simulink model "TEP_Final_NoScript"  (R2024a)
settings: Solver=FixedStepAuto  StartTime=0.0  StopTime=10  FixedStep=1/3600  RelTol=1e-3
model workspace (MAT data in the model file):
  AD : Simulink.Parameter (value not decoded)
  AG : Simulink.Parameter (value not decoded)
  AH : Simulink.Parameter (value not decoded)
  AV : Simulink.Parameter (value not decoded)
  AVP : Simulink.Parameter (value not decoded)
  BCHL : Simulink.Parameter (value not decoded)
  BCHV : Simulink.Parameter (value not decoded)
  BD : Simulink.Parameter (value not decoded)
  BG : Simulink.Parameter (value not decoded)
  BH : Simulink.Parameter (value not decoded)
  BVP : Simulink.Parameter (value not decoded)
  CD : Simulink.Parameter (value not decoded)
  CG : Simulink.Parameter (value not decoded)
  CH : Simulink.Parameter (value not decoded)
  CVP : Simulink.Parameter (value not decoded)
  XMW : Simulink.Parameter (value not decoded)
  XNS : Simulink.Parameter (value not decoded)
  XNSE : Simulink.Parameter (value not decoded)
symbols that are objects in the model workspace (value not decoded): AD, AG, AH, AV, AVP, BD, BG, BH, BVP, CD, CG, CH, CVP, XMW, XNS, XNSE
undefined symbols (not defined in the file or in its folder): magnitude, msgbox, SETPT, XMEAS, XMV
libraries: mylib x360, dspindex x28
(part 10 of 14)

== system TEP_Final_NoScript/Subsystem/Braatz/ 10/CONTROL 6 ==
  SETPT(6) : Inport
  XMEAS : Inport  Port=2
  Constant1 : Constant  Value=GAIN6
  Constant2 : Constant  Value=HIGH6
  Constant3 : Constant  Value=SI6
  Constant4 : Constant  Value=XMV6_0
  P Control : Subsystem
  Sampling interval : mylib/Braatz Control/Sampling interval  SystemSampleTime=-1  VariantActivationTime=update diagram  AllowFlexibleInterface=on  Latency=0  AutoFrameSizeCalculation=off
      settings: SourceProductName=TEP Library
  XMV(6) : Outport  VectorParamsAs1DForOutWhenUnconnected=off
  wires:
  Constant2/1 -> P Control/4(High Limit)
  Constant1/1 -> P Control/2(GAIN)
  SETPT(6)/1 -> P Control/1(SETPT)
  P Control/1(XMV_NEW) -> XMV(6)/1
  Sampling interval/1 -> P Control/Action
  Constant3/1 -> Sampling interval/1
  XMEAS/1 -> P Control/3(XMEAS)
  Constant4/1 -> P Control/5(XMV_0)

== system TEP_Final_NoScript/Subsystem/Braatz/ 2/CONTROL 13 ==
  XMEAS(23) : Inport
  Constant : Constant  Value=SETPT13
  Constant1 : Constant  Value=GAIN13
  Constant2 : Constant  Value=TAUI13
  Constant3 : Constant  Value=HIGH13
  Constant5 : Constant  Value=SI13
  Constant6 : Constant  Value=HIGH3
  PI Control Setpoint : mylib/Braatz Control/PI Control Setpoint  SystemSampleTime=-1  VariantActivationTime=update diagram  AllowFlexibleInterface=on  Latency=0  AutoFrameSizeCalculation=off
      settings: SourceProductName=TEP Library
  SETPT_0 : Constant  Value=SETPT3
  Sampling interval : mylib/Braatz Control/Sampling interval  SystemSampleTime=-1  VariantActivationTime=update diagram  AllowFlexibleInterface=on  Latency=0  AutoFrameSizeCalculation=off
      settings: SourceProductName=TEP Library
  SETPT(3) : Outport  VectorParamsAs1DForOutWhenUnconnected=off
  wires:
  Sampling interval/1 -> PI Control Setpoint/Action
  Constant/1 -> PI Control Setpoint/1
  XMEAS(23)/1 -> PI Control Setpoint/2
  PI Control Setpoint/1 -> SETPT(3)/1
  Constant2/1 -> PI Control Setpoint/7
  Constant5/1 -> PI Control Setpoint/6, Sampling interval/1
  Constant1/1 -> PI Control Setpoint/5
  Constant3/1 -> PI Control Setpoint/3
  Constant6/1 -> PI Control Setpoint/4
  SETPT_0/1 -> PI Control Setpoint/8

== system TEP_Final_NoScript/Subsystem/Braatz/ 2/CONTROL 3 ==
  XMEAS(1) : Inport
  SETPT(3) : Inport  Port=2
  Constant1 : Constant  Value=GAIN3
  Constant2 : Constant  Value=HIGH3
  Constant3 : Constant  Value=SI3
  Constant4 : Constant  Value=XMV3_0
  Display2 : Display
  P Control : mylib/Braatz Control/P Control  SystemSampleTime=-1  VariantActivationTime=update diagram  AllowFlexibleInterface=on  Latency=0  AutoFrameSizeCalculation=off
      settings: SourceProductName=TEP Library
  Sampling interval : mylib/Braatz Control/Sampling interval  SystemSampleTime=-1  VariantActivationTime=update diagram  AllowFlexibleInterface=on  Latency=0  AutoFrameSizeCalculation=off
      settings: SourceProductName=TEP Library
  XMV(3) : Outport
  wires:
  Constant2/1 -> P Control/4
  Constant1/1 -> P Control/2
  XMEAS(1)/1 -> Display2/1, P Control/3
  Sampling interval/1 -> P Control/Action
  Constant3/1 -> Sampling interval/1
  Constant4/1 -> P Control/5
  P Control/1 -> XMV(3)/1
  SETPT(3)/1 -> P Control/1

== system TEP_Final_NoScript/Subsystem/Braatz/ 3/CONTROL 17 ==
  XMEAS(8) : Inport
  Constant : Constant  Value=SETPT17
  Constant1 : Constant  Value=GAIN17
  Constant2 : Constant  Value=TAUI17
  Constant3 : Constant  Value=HIGH17
  Constant4 : Constant  Value=SETPT4
  Constant5 : Constant  Value=SI17
  Constant6 : Constant  Value=HIGH4
  PI Control Setpoint : mylib/Braatz Control/PI Control Setpoint  SystemSampleTime=-1  VariantActivationTime=update diagram  AllowFlexibleInterface=on  Latency=0  AutoFrameSizeCalculation=off
      settings: SourceProductName=TEP Library
  Sampling interval : mylib/Braatz Control/Sampling interval  SystemSampleTime=-1  VariantActivationTime=update diagram  AllowFlexibleInterface=on  Latency=0  AutoFrameSizeCalculation=off
      settings: SourceProductName=TEP Library
  SETPT(4) : Outport  VectorParamsAs1DForOutWhenUnconnected=off
  wires:
  Sampling interval/1 -> PI Control Setpoint/Action
  Constant/1 -> PI Control Setpoint/1
  XMEAS(8)/1 -> PI Control Setpoint/2
  PI Control Setpoint/1 -> SETPT(4)/1
  Constant5/1 -> PI Control Setpoint/6, Sampling interval/1
  Constant3/1 -> PI Control Setpoint/3
  Constant6/1 -> PI Control Setpoint/4
  Constant1/1 -> PI Control Setpoint/5
  Constant2/1 -> PI Control Setpoint/7
  Constant4/1 -> PI Control Setpoint/8

== system TEP_Final_NoScript/Subsystem/Braatz/ 3/CONTROL 4 ==
  XMEAS(4) : Inport
  SETPT(4) : Inport  Port=2
  Constant1 : Constant  Value=GAIN4
  Constant2 : Constant  Value=HIGH4
  Constant3 : Constant  Value=SI4
  Constant4 : Constant  Value=XMV4_0
  P Control : mylib/Braatz Control/P Control  SystemSampleTime=-1  VariantActivationTime=update diagram  AllowFlexibleInterface=on  Latency=0  AutoFrameSizeCalculation=off
      settings: SourceProductName=TEP Library
  Sampling interval : mylib/Braatz Control/Sampling interval  SystemSampleTime=-1  VariantActivationTime=update diagram  AllowFlexibleInterface=on  Latency=0  AutoFrameSizeCalculation=off
      settings: SourceProductName=TEP Library
  XMV(4) : Outport  VectorParamsAs1DForOutWhenUnconnected=off
  wires:
  SETPT(4)/1 -> P Control/1
  P Control/1 -> XMV(4)/1
  Sampling interval/1 -> P Control/Action
  Constant3/1 -> Sampling interval/1
  XMEAS(4)/1 -> P Control/3
  Constant1/1 -> P Control/2
  Constant4/1 -> P Control/5
  Constant2/1 -> P Control/4

== system TEP_Final_NoScript/Subsystem/Braatz/ 4/CONTROL 5 ==
  XMEAS(5) : Inport
  Constant1 : Constant  Value=GAIN5
  Constant2 : Constant  Value=HIGH5
  Constant3 : Constant  Value=SI5
  Constant4 : Constant  Value=SETPT5
  Constant5 : Constant  Value=TAUI5
  Constant6 : Constant  Value=XMV5_0
  PI Control : mylib/Braatz Control/PI Control  SystemSampleTime=-1  VariantActivationTime=update diagram  AllowFlexibleInterface=on  Latency=0  AutoFrameSizeCalculation=off
      settings: SourceProductName=TEP Library
  Sampling interval : mylib/Braatz Control/Sampling interval  SystemSampleTime=-1  VariantActivationTime=update diagram  AllowFlexibleInterface=on  Latency=0  AutoFrameSizeCalculation=off
      settings: SourceProductName=TEP Library
  XMV(5) : Outport  VectorParamsAs1DForOutWhenUnconnected=off
  wires:
  Constant2/1 -> PI Control/3
  Constant1/1 -> PI Control/4
  XMEAS(5)/1 -> PI Control/2
  PI Control/1 -> XMV(5)/1
  Sampling interval/1 -> PI Control/Action
  Constant3/1 -> PI Control/5, Sampling interval/1
  Constant4/1 -> PI Control/1
  Constant5/1 -> PI Control/6
  Constant6/1 -> PI Control/7

== system TEP_Final_NoScript/Subsystem/Braatz/ 5/CONTROL 7 ==
  XMEAS(12) : Inport
  Constant1 : Constant  Value=GAIN7
  Constant2 : Constant  Value=HIGH7
  Constant3 : Constant  Value=SI7
  Constant4 : Constant  Value=SETPT7
  Constant5 : Constant  Value=XMV7_0
  P Control : mylib/Braatz Control/P Control  SystemSampleTime=-1  VariantActivationTime=update diagram  AllowFlexibleInterface=on  Latency=0  AutoFrameSizeCalculation=off
      settings: SourceProductName=TEP Library
  Sampling interval : mylib/Braatz Control/Sampling interval  SystemSampleTime=-1  VariantActivationTime=update diagram  AllowFlexibleInterface=on  Latency=0  AutoFrameSizeCalculation=off
      settings: SourceProductName=TEP Library
  XMV(7) : Outport  VectorParamsAs1DForOutWhenUnconnected=off
  wires:
  P Control/1 -> XMV(7)/1
  Sampling interval/1 -> P Control/Action
  Constant3/1 -> Sampling interval/1
  Constant4/1 -> P Control/1
  Constant2/1 -> P Control/4
  XMEAS(12)/1 -> P Control/3
  Constant1/1 -> P Control/2
  Constant5/1 -> P Control/5

== system TEP_Final_NoScript/Subsystem/Braatz/ 6/CONTROL 8 ==
  XMEAS(15) : Inport
  Constant1 : Constant  Value=GAIN8
  Constant2 : Constant  Value=HIGH8
  Constant3 : Constant  Value=SI8
  Constant4 : Constant  Value=SETPT8
  Constant5 : Constant  Value=XMV8_0
  P Control : mylib/Braatz Control/P Control  SystemSampleTime=-1  VariantActivationTime=update diagram  AllowFlexibleInterface=on  Latency=0  AutoFrameSizeCalculation=off
      settings: SourceProductName=TEP Library
  Sampling interval : mylib/Braatz Control/Sampling interval  SystemSampleTime=-1  VariantActivationTime=update diagram  AllowFlexibleInterface=on  Latency=0  AutoFrameSizeCalculation=off
      settings: SourceProductName=TEP Library
  XMV(8) : Outport  VectorParamsAs1DForOutWhenUnconnected=off
  wires:
  P Control/1 -> XMV(8)/1
  Sampling interval/1 -> P Control/Action
  Constant3/1 -> Sampling interval/1
  Constant4/1 -> P Control/1
  Constant2/1 -> P Control/4
  XMEAS(15)/1 -> P Control/3
  Constant1/1 -> P Control/2
  Constant5/1 -> P Control/5

== system TEP_Final_NoScript/Subsystem/Braatz/ 7/CONTROL 11 ==
  XMEAS(17) : Inport
  Constant1 : Constant  Value=GAIN11
  Constant2 : Constant  Value=HIGH11
  Constant3 : Constant  Value=SI11
  Constant4 : Constant  Value=SETPT11
  Constant5 : Constant  Value=TAUI11
  Constant6 : Constant  Value=XMV11_0
  PI Control : mylib/Braatz Control/PI Control  SystemSampleTime=-1  VariantActivationTime=update diagram  AllowFlexibleInterface=on  Latency=0  AutoFrameSizeCalculation=off
      settings: SourceProductName=TEP Library
  Sampling interval : mylib/Braatz Control/Sampling interval  SystemSampleTime=-1  VariantActivationTime=update diagram  AllowFlexibleInterface=on  Latency=0  AutoFrameSizeCalculation=off
      settings: SourceProductName=TEP Library
  XMV(11) : Outport  VectorParamsAs1DForOutWhenUnconnected=off
  wires:
  PI Control/1 -> XMV(11)/1
  Sampling interval/1 -> PI Control/Action
  Constant3/1 -> PI Control/5, Sampling interval/1
  Constant4/1 -> PI Control/1
  XMEAS(17)/1 -> PI Control/2
  Constant2/1 -> PI Control/3
  Constant1/1 -> PI Control/4
  Constant5/1 -> PI Control/6
  Constant6/1 -> PI Control/7

== system TEP_Final_NoScript/Subsystem/Braatz/ 8/CONTROL 10 ==
  XMEAS(21) : Inport
  SETPT(10) : Inport  Port=2
  Constant1 : Constant  Value=GAIN10
  Constant2 : Constant  Value=HIGH10
  Constant3 : Constant  Value=SI10
  Constant4 : Constant  Value=TAUI10
  Constant5 : Constant  Value=XMV10_0
  PI Control : mylib/Braatz Control/PI Control  SystemSampleTime=-1  VariantActivationTime=update diagram  AllowFlexibleInterface=on  Latency=0  AutoFrameSizeCalculation=off
      settings: SourceProductName=TEP Library
  Sampling interval : mylib/Braatz Control/Sampling interval  SystemSampleTime=-1  VariantActivationTime=update diagram  AllowFlexibleInterface=on  Latency=0  AutoFrameSizeCalculation=off
      settings: SourceProductName=TEP Library
  XMV(10) : Outport  VectorParamsAs1DForOutWhenUnconnected=off
  wires:
  PI Control/1 -> XMV(10)/1
  Sampling interval/1 -> PI Control/Action
  Constant3/1 -> PI Control/5, Sampling interval/1
  SETPT(10)/1 -> PI Control/1
  XMEAS(21)/1 -> PI Control/2
  Constant2/1 -> PI Control/3
  Constant1/1 -> PI Control/4
  Constant4/1 -> PI Control/6
  Constant5/1 -> PI Control/7

== system TEP_Final_NoScript/Subsystem/Braatz/ 8/CONTROL 18 ==
  XMEAS(9) : Inport
  Constant : Constant  Value=SETPT18
  Constant1 : Constant  Value=GAIN18
  Constant2 : Constant  Value=TAUI18
  Constant3 : Constant  Value=HIGH18
  Constant4 : Constant  Value=SETPT10
  Constant5 : Constant  Value=SI18
  Constant6 : Constant  Value=HIGH10
  PI Control Setpoint : mylib/Braatz Control/PI Control Setpoint  SystemSampleTime=-1  VariantActivationTime=update diagram  AllowFlexibleInterface=on  Latency=0  AutoFrameSizeCalculation=off
      settings: SourceProductName=TEP Library
  Sampling interval : mylib/Braatz Control/Sampling interval  SystemSampleTime=-1  VariantActivationTime=update diagram  AllowFlexibleInterface=on  Latency=0  AutoFrameSizeCalculation=off
      settings: SourceProductName=TEP Library
  SETPT(10) : Outport  VectorParamsAs1DForOutWhenUnconnected=off
  wires:
  Sampling interval/1 -> PI Control Setpoint/Action
  Constant/1 -> PI Control Setpoint/1
  XMEAS(9)/1 -> PI Control Setpoint/2
  PI Control Setpoint/1 -> SETPT(10)/1
  Constant5/1 -> PI Control Setpoint/6, Sampling interval/1
  Constant3/1 -> PI Control Setpoint/3
  Constant6/1 -> PI Control Setpoint/4
  Constant1/1 -> PI Control Setpoint/5
  Constant2/1 -> PI Control Setpoint/7
  Constant4/1 -> PI Control Setpoint/8

== system TEP_Final_NoScript/Subsystem/Braatz/ 9/CONTROL 16 ==
  XMEAS(18) : Inport
  SETPT(16) : Inport  Port=2
  Constant1 : Constant  Value=GAIN16
  Constant2 : Constant  Value=TAUI16
  Constant3 : Constant  Value=HIGH16
  Constant4 : Constant  Value=SETPT9
  Constant5 : Constant  Value=SI16
  Constant6 : Constant  Value=HIGH9
  PI Control Setpoint : mylib/Braatz Control/PI Control Setpoint  SystemSampleTime=-1  VariantActivationTime=update diagram  AllowFlexibleInterface=on  Latency=0  AutoFrameSizeCalculation=off
      settings: SourceProductName=TEP Library
  Sampling interval : mylib/Braatz Control/Sampling interval  SystemSampleTime=-1  VariantActivationTime=update diagram  AllowFlexibleInterface=on  Latency=0  AutoFrameSizeCalculation=off
      settings: SourceProductName=TEP Library
  SETPT(9) : Outport  VectorParamsAs1DForOutWhenUnconnected=off
  wires:
  Sampling interval/1 -> PI Control Setpoint/Action
  SETPT(16)/1 -> PI Control Setpoint/1
  XMEAS(18)/1 -> PI Control Setpoint/2
  PI Control Setpoint/1 -> SETPT(9)/1
  Constant5/1 -> PI Control Setpoint/6, Sampling interval/1
  Constant3/1 -> PI Control Setpoint/3
  Constant6/1 -> PI Control Setpoint/4
  Constant1/1 -> PI Control Setpoint/5
  Constant2/1 -> PI Control Setpoint/7
  Constant4/1 -> PI Control Setpoint/8

== system TEP_Final_NoScript/Subsystem/Braatz/ 9/CONTROL 20 ==
  XMEAS(38) : Inport
  Constant : Constant  Value=SETPT20
  Constant1 : Constant  Value=GAIN20
  Constant2 : Constant  Value=TAUI20
  Constant3 : Constant  Value=HIGH20
  Constant4 : Constant  Value=SETPT16
  Constant5 : Constant  Value=SI20
  Constant6 : Constant  Value=HIGH16
  PI Control Setpoint : mylib/Braatz Control/PI Control Setpoint  SystemSampleTime=-1  VariantActivationTime=update diagram  AllowFlexibleInterface=on  Latency=0  AutoFrameSizeCalculation=off
      settings: SourceProductName=TEP Library
  Sampling interval : mylib/Braatz Control/Sampling interval  SystemSampleTime=-1  VariantActivationTime=update diagram  AllowFlexibleInterface=on  Latency=0  AutoFrameSizeCalculation=off
      settings: SourceProductName=TEP Library
  SETPT(16) : Outport  VectorParamsAs1DForOutWhenUnconnected=off
  wires:
  Sampling interval/1 -> PI Control Setpoint/Action
  Constant/1 -> PI Control Setpoint/1
  XMEAS(38)/1 -> PI Control Setpoint/2
  PI Control Setpoint/1 -> SETPT(16)/1
  Constant5/1 -> PI Control Setpoint/6, Sampling interval/1
  Constant3/1 -> PI Control Setpoint/3
  Constant6/1 -> PI Control Setpoint/4
  Constant1/1 -> PI Control Setpoint/5
  Constant2/1 -> PI Control Setpoint/7
  Constant4/1 -> PI Control Setpoint/8

== system TEP_Final_NoScript/Subsystem/Braatz/ 9/CONTROL 9 ==
  XMEAS(19) : Inport
  SETPT(9) : Inport  Port=2
  Constant1 : Constant  Value=GAIN9
  Constant2 : Constant  Value=HIGH9
  Constant3 : Constant  Value=SI9
  Constant4 : Constant  Value=XMV9_0
  P Control : mylib/Braatz Control/P Control  SystemSampleTime=-1  VariantActivationTime=update diagram  AllowFlexibleInterface=on  Latency=0  AutoFrameSizeCalculation=off
      settings: SourceProductName=TEP Library
  Sampling interval : mylib/Braatz Control/Sampling interval  SystemSampleTime=-1  VariantActivationTime=update diagram  AllowFlexibleInterface=on  Latency=0  AutoFrameSizeCalculation=off
      settings: SourceProductName=TEP Library
  XMV(9) : Outport  VectorParamsAs1DForOutWhenUnconnected=off
  wires:
  SETPT(9)/1 -> P Control/1
  P Control/1 -> XMV(9)/1
  Sampling interval/1 -> P Control/Action
  Constant3/1 -> Sampling interval/1
  XMEAS(19)/1 -> P Control/3
  Constant1/1 -> P Control/2
  Constant2/1 -> P Control/4
  Constant4/1 -> P Control/5

== system TEP_Final_NoScript/Subsystem1/A and C feed stream/Composition measurement mol%/Subsystem ==
  XST : Inport
  XMNSE : Inport  Port=2
  Bus Selector : BusSelector  OutputSignals=XMNSEA,XMNSEB,XMNSEC,XMNSED,XMNSEE,XMNSEF,XMNSEG,XMNSEH
  Process Noise I=23-{1..7,36} (8 alike) : mylib/Process Noise I=23-36  SystemSampleTime=-1  VariantActivationTime=update diagram  AllowFlexibleInterface=on  Latency=0  AutoFrameSizeCalculation=off
      settings: SourceProductName=TEP Library
  Subsystem : Subsystem
  SMEASXA : Outport  VectorParamsAs1DForOutWhenUnconnected=off
  SMEASXB : Outport  Port=2  VectorParamsAs1DForOutWhenUnconnected=off
  SMEASXC : Outport  Port=3  VectorParamsAs1DForOutWhenUnconnected=off
  SMEASXD : Outport  Port=4  VectorParamsAs1DForOutWhenUnconnected=off
  SMEASXE : Outport  Port=5  VectorParamsAs1DForOutWhenUnconnected=off
  SMEASXF : Outport  Port=6  VectorParamsAs1DForOutWhenUnconnected=off
  SMEASXG : Outport  Port=7  VectorParamsAs1DForOutWhenUnconnected=off
  SMEASXH : Outport  Port=8  VectorParamsAs1DForOutWhenUnconnected=off
  wires:
  Process Noise I=23-36/1 -> SMEASXA/1
  Process Noise I=23-1/1 -> SMEASXB/1
  Bus Selector/2 -> Process Noise I=23-1/2  "<XMNSEB>"
  Process Noise I=23-2/1 -> SMEASXC/1
  Process Noise I=23-3/1 -> SMEASXD/1
  Process Noise I=23-4/1 -> SMEASXE/1
  Process Noise I=23-5/1 -> SMEASXF/1
  Process Noise I=23-6/1 -> SMEASXG/1
  Process Noise I=23-7/1 -> SMEASXH/1
  Bus Selector/7 -> Process Noise I=23-6/2  "<XMNSEG>"
  Bus Selector/8 -> Process Noise I=23-7/2  "<XMNSEH>"
  Bus Selector/6 -> Process Noise I=23-5/2  "<XMNSEF>"
  Bus Selector/5 -> Process Noise I=23-4/2  "<XMNSEE>"
  Bus Selector/4 -> Process Noise I=23-3/2  "<XMNSED>"
  Bus Selector/3 -> Process Noise I=23-2/2  "<XMNSEC>"
  Bus Selector/1 -> Process Noise I=23-36/2  "<XMNSEA>"
  XST/1 -> Subsystem/1(XST)
  Subsystem/1(XCMPA) -> Process Noise I=23-36/1
  Subsystem/2(XCMPB) -> Process Noise I=23-1/1
  Subsystem/3(XCMPC) -> Process Noise I=23-2/1
  Subsystem/4(XCMPD) -> Process Noise I=23-3/1
  Subsystem/5("XCMPE ") -> Process Noise I=23-4/1
  Subsystem/6("XCMPF ") -> Process Noise I=23-5/1
  Subsystem/7(XCMPG) -> Process Noise I=23-6/1
  Subsystem/8("XCMPH ") -> Process Noise I=23-7/1
  XMNSE/1 -> Bus Selector/1

== system TEP_Final_NoScript/Subsystem1/A and C feed stream/Flow measurement in kg//h/XMWS Molecular weight of Stream lb//lb-mol ==
  XST : Inport
  Product : Product
  Sum of Elements : Sum  Inputs=+
  "XMW(I) Molecular weight of components lb/lb-mol " : Constant  Value=XMW
  XMWS : Outport  VectorParamsAs1DForOutWhenUnconnected=off
  wires:
  Sum of Elements/1 -> XMWS/1
  Product/1 -> Sum of Elements/1
  XST/1 -> Product/1
  "XMW(I) Molecular weight of components lb/lb-mol "/1 -> Product/2

== system TEP_Final_NoScript/Subsystem1/A feed stream/Composition measurement mol%/Subsystem ==
  XST : Inport
  XMNSE : Inport  Port=2
  Bus Selector : BusSelector  OutputSignals=XMNSEA,XMNSEB,XMNSEC,XMNSED,XMNSEE,XMNSEF,XMNSEG,XMNSEH
  Process Noise I=23-{1..7,36} (8 alike) : mylib/Process Noise I=23-36  SystemSampleTime=-1  VariantActivationTime=update diagram  AllowFlexibleInterface=on  Latency=0  AutoFrameSizeCalculation=off
      settings: SourceProductName=TEP Library
  Subsystem : Subsystem
  SMEASXA : Outport  VectorParamsAs1DForOutWhenUnconnected=off
  SMEASXB : Outport  Port=2  VectorParamsAs1DForOutWhenUnconnected=off
  SMEASXC : Outport  Port=3  VectorParamsAs1DForOutWhenUnconnected=off
  SMEASXD : Outport  Port=4  VectorParamsAs1DForOutWhenUnconnected=off
  SMEASXE : Outport  Port=5  VectorParamsAs1DForOutWhenUnconnected=off
  SMEASXF : Outport  Port=6  VectorParamsAs1DForOutWhenUnconnected=off
  SMEASXG : Outport  Port=7  VectorParamsAs1DForOutWhenUnconnected=off
  SMEASXH : Outport  Port=8  VectorParamsAs1DForOutWhenUnconnected=off
  wires:
  Process Noise I=23-36/1 -> SMEASXA/1
  Process Noise I=23-1/1 -> SMEASXB/1
  Bus Selector/2 -> Process Noise I=23-1/2  "<XMNSEB>"
  Process Noise I=23-2/1 -> SMEASXC/1
  Process Noise I=23-3/1 -> SMEASXD/1
  Process Noise I=23-4/1 -> SMEASXE/1
  Process Noise I=23-5/1 -> SMEASXF/1
  Process Noise I=23-6/1 -> SMEASXG/1
  Process Noise I=23-7/1 -> SMEASXH/1
  Bus Selector/7 -> Process Noise I=23-6/2  "<XMNSEG>"
  Bus Selector/8 -> Process Noise I=23-7/2  "<XMNSEH>"
  Bus Selector/6 -> Process Noise I=23-5/2  "<XMNSEF>"
  Bus Selector/5 -> Process Noise I=23-4/2  "<XMNSEE>"
  Bus Selector/4 -> Process Noise I=23-3/2  "<XMNSED>"
  Bus Selector/3 -> Process Noise I=23-2/2  "<XMNSEC>"
  Bus Selector/1 -> Process Noise I=23-36/2  "<XMNSEA>"
  XST/1 -> Subsystem/1(XST)
  Subsystem/1(XCMPA) -> Process Noise I=23-36/1
  Subsystem/2(XCMPB) -> Process Noise I=23-1/1
  Subsystem/3(XCMPC) -> Process Noise I=23-2/1
  Subsystem/4(XCMPD) -> Process Noise I=23-3/1
  Subsystem/5("XCMPE ") -> Process Noise I=23-4/1
  Subsystem/6("XCMPF ") -> Process Noise I=23-5/1
  Subsystem/7(XCMPG) -> Process Noise I=23-6/1
  Subsystem/8("XCMPH ") -> Process Noise I=23-7/1
  XMNSE/1 -> Bus Selector/1

== system TEP_Final_NoScript/Subsystem1/A feed stream/Flow measurement in kg//h/XMWS Molecular weight of Stream lb//lb-mol ==
  XST : Inport
  Product : Product
  Sum of Elements : Sum  Inputs=+
  "XMW(I) Molecular weight of components lb/lb-mol " : Constant  Value=XMW
  XMWS : Outport  VectorParamsAs1DForOutWhenUnconnected=off
  wires:
  Sum of Elements/1 -> XMWS/1
  Product/1 -> Sum of Elements/1
  XST/1 -> Product/1
  "XMW(I) Molecular weight of components lb/lb-mol "/1 -> Product/2

== system TEP_Final_NoScript/Subsystem1/CCin/Subsystem3/Subsystem ==
  T1 : Inport
  T0 : Inport  Port=2
  Product3 : Product
  Subsystem2 : Subsystem
  Universal gas constant J/molK : Constant  Value=8.314
  h-h0 J/mol : Outport
  wires:
  T1/1 -> Subsystem2/1(T1)
  T0/1 -> Subsystem2/2(T0)
  Subsystem2/1(AT) -> Product3/1
  Universal gas constant J/molK/1 -> Product3/2
  Product3/1 -> h-h0 J/mol/1

== system TEP_Final_NoScript/Subsystem1/CCin/Subsystem3/Subsystem1 ==
  T1 : Inport
  T0 : Inport  Port=2
  P1 : Inport  Port=3
  P0 : Inport  Port=4
  " " : Product
  Add : Sum  Inputs=+-
  Display{1..8} (8 alike) : Display
  Divide : Product  Inputs=*/
  Math Function2 : Math  Operator=log  SignedPower=on
  Product3 : Product  Inputs=3
  Product6 : Product
  Subsystem : Subsystem
  Universal gas constant J/molK : Constant  Value=8.314
  T0(s-s0) J/mol : Outport
  wires:
  T1/1 -> Display6/1, Subsystem/1(T1)
  Subsystem/1(AT) -> Display8/1, Product3/1
  Universal gas constant J/molK/1 -> Product6/1, Product3/2
  T0/1 -> " "/1, Display7/1, Product3/3, Subsystem/2(T0)
  Math Function2/1 -> Display5/1, Product6/2
  Product6/1 -> Display4/1, " "/2
  Divide/1 -> Display2/1, Math Function2/1
  P0/1 -> Divide/2
  P1/1 -> Divide/1
  Product3/1 -> Add/1, Display3/1
  Add/1 -> T0(s-s0) J/mol/1
  " "/1 -> Add/2, Display1/1

== system TEP_Final_NoScript/Subsystem1/CCin/Subsystem3/Subsystem2 ==
  TC : Inport
  Temperature in Kelvin K : Sum
  To Convert °C to K : Constant  Value=273.15
  TK : Outport
  wires:
  TC/1 -> Temperature in Kelvin K/1
  Temperature in Kelvin K/1 -> TK/1
  To Convert °C to K/1 -> Temperature in Kelvin K/2

== system TEP_Final_NoScript/Subsystem1/CCout/Subsystem3/Subsystem ==
  T1 : Inport
  T0 : Inport  Port=2
  Product3 : Product
  Subsystem2 : Subsystem
  Universal gas constant J/molK : Constant  Value=8.314
  h-h0 J/mol : Outport
  wires:
  T1/1 -> Subsystem2/1(T1)
  T0/1 -> Subsystem2/2(T0)
  Subsystem2/1(AT) -> Product3/1
  Universal gas constant J/molK/1 -> Product3/2
  Product3/1 -> h-h0 J/mol/1

== system TEP_Final_NoScript/Subsystem1/CCout/Subsystem3/Subsystem1 ==
  T1 : Inport
  T0 : Inport  Port=2
  P1 : Inport  Port=3
  P0 : Inport  Port=4
  " " : Product
  Add : Sum  Inputs=+-
  Display{1..8} (8 alike) : Display
  Divide : Product  Inputs=*/
  Math Function2 : Math  Operator=log  SignedPower=on
  Product3 : Product  Inputs=3
  Product6 : Product
  Subsystem : Subsystem
  Universal gas constant J/molK : Constant  Value=8.314
  T0(s-s0) J/mol : Outport
  wires:
  T1/1 -> Display6/1, Subsystem/1(T1)
  Subsystem/1(AT) -> Display8/1, Product3/1
  Universal gas constant J/molK/1 -> Product6/1, Product3/2
  T0/1 -> " "/1, Display7/1, Product3/3, Subsystem/2(T0)
  Math Function2/1 -> Display5/1, Product6/2
  Product6/1 -> Display4/1, " "/2
  Divide/1 -> Display2/1, Math Function2/1
  P0/1 -> Divide/2
  P1/1 -> Divide/1
  Product3/1 -> Add/1, Display3/1
  Add/1 -> T0(s-s0) J/mol/1
  " "/1 -> Add/2, Display1/1

== system TEP_Final_NoScript/Subsystem1/CCout/Subsystem3/Subsystem2 ==
  TC : Inport
  Temperature in Kelvin K : Sum
  To Convert °C to K : Constant  Value=273.15
  TK : Outport
  wires:
  TC/1 -> Temperature in Kelvin K/1
  Temperature in Kelvin K/1 -> TK/1
  To Convert °C to K/1 -> Temperature in Kelvin K/2

== system TEP_Final_NoScript/Subsystem1/D feed stream/Composition measurement mol%/Subsystem ==
  XST : Inport
  XMNSE : Inport  Port=2
  Bus Selector : BusSelector  OutputSignals=XMNSEA,XMNSEB,XMNSEC,XMNSED,XMNSEE,XMNSEF,XMNSEG,XMNSEH
  Process Noise I=23-{1..7,36} (8 alike) : mylib/Process Noise I=23-36  SystemSampleTime=-1  VariantActivationTime=update diagram  AllowFlexibleInterface=on  Latency=0  AutoFrameSizeCalculation=off
      settings: SourceProductName=TEP Library
  Subsystem : Subsystem
  SMEASXA : Outport  VectorParamsAs1DForOutWhenUnconnected=off
  SMEASXB : Outport  Port=2  VectorParamsAs1DForOutWhenUnconnected=off
  SMEASXC : Outport  Port=3  VectorParamsAs1DForOutWhenUnconnected=off
  SMEASXD : Outport  Port=4  VectorParamsAs1DForOutWhenUnconnected=off
  SMEASXE : Outport  Port=5  VectorParamsAs1DForOutWhenUnconnected=off
  SMEASXF : Outport  Port=6  VectorParamsAs1DForOutWhenUnconnected=off
  SMEASXG : Outport  Port=7  VectorParamsAs1DForOutWhenUnconnected=off
  SMEASXH : Outport  Port=8  VectorParamsAs1DForOutWhenUnconnected=off
  wires:
  Process Noise I=23-36/1 -> SMEASXA/1
  Process Noise I=23-1/1 -> SMEASXB/1
  Bus Selector/2 -> Process Noise I=23-1/2  "<XMNSEB>"
  Process Noise I=23-2/1 -> SMEASXC/1
  Process Noise I=23-3/1 -> SMEASXD/1
  Process Noise I=23-4/1 -> SMEASXE/1
  Process Noise I=23-5/1 -> SMEASXF/1
  Process Noise I=23-6/1 -> SMEASXG/1
  Process Noise I=23-7/1 -> SMEASXH/1
  Bus Selector/7 -> Process Noise I=23-6/2  "<XMNSEG>"
  Bus Selector/8 -> Process Noise I=23-7/2  "<XMNSEH>"
  Bus Selector/6 -> Process Noise I=23-5/2  "<XMNSEF>"
  Bus Selector/5 -> Process Noise I=23-4/2  "<XMNSEE>"
  Bus Selector/4 -> Process Noise I=23-3/2  "<XMNSED>"
  Bus Selector/3 -> Process Noise I=23-2/2  "<XMNSEC>"
  Bus Selector/1 -> Process Noise I=23-36/2  "<XMNSEA>"
  XST/1 -> Subsystem/1(XST)
  Subsystem/1(XCMPA) -> Process Noise I=23-36/1
  Subsystem/2(XCMPB) -> Process Noise I=23-1/1
  Subsystem/3(XCMPC) -> Process Noise I=23-2/1
  Subsystem/4(XCMPD) -> Process Noise I=23-3/1
  Subsystem/5("XCMPE ") -> Process Noise I=23-4/1
  Subsystem/6("XCMPF ") -> Process Noise I=23-5/1
  Subsystem/7(XCMPG) -> Process Noise I=23-6/1
  Subsystem/8("XCMPH ") -> Process Noise I=23-7/1
  XMNSE/1 -> Bus Selector/1

== system TEP_Final_NoScript/Subsystem1/E feed stream/Composition measurement mol%/Subsystem ==
  XST : Inport
  XMNSE : Inport  Port=2
  Bus Selector : BusSelector  OutputSignals=XMNSEA,XMNSEB,XMNSEC,XMNSED,XMNSEE,XMNSEF,XMNSEG,XMNSEH
  Process Noise I=23-{1..7,36} (8 alike) : mylib/Process Noise I=23-36  SystemSampleTime=-1  VariantActivationTime=update diagram  AllowFlexibleInterface=on  Latency=0  AutoFrameSizeCalculation=off
      settings: SourceProductName=TEP Library
  Subsystem : Subsystem
  SMEASXA : Outport  VectorParamsAs1DForOutWhenUnconnected=off
  SMEASXB : Outport  Port=2  VectorParamsAs1DForOutWhenUnconnected=off
  SMEASXC : Outport  Port=3  VectorParamsAs1DForOutWhenUnconnected=off
  SMEASXD : Outport  Port=4  VectorParamsAs1DForOutWhenUnconnected=off
  SMEASXE : Outport  Port=5  VectorParamsAs1DForOutWhenUnconnected=off
  SMEASXF : Outport  Port=6  VectorParamsAs1DForOutWhenUnconnected=off
  SMEASXG : Outport  Port=7  VectorParamsAs1DForOutWhenUnconnected=off
  SMEASXH : Outport  Port=8  VectorParamsAs1DForOutWhenUnconnected=off
  wires:
  Process Noise I=23-36/1 -> SMEASXA/1
  Process Noise I=23-1/1 -> SMEASXB/1
  Bus Selector/2 -> Process Noise I=23-1/2  "<XMNSEB>"
  Process Noise I=23-2/1 -> SMEASXC/1
  Process Noise I=23-3/1 -> SMEASXD/1
  Process Noise I=23-4/1 -> SMEASXE/1
  Process Noise I=23-5/1 -> SMEASXF/1
  Process Noise I=23-6/1 -> SMEASXG/1
  Process Noise I=23-7/1 -> SMEASXH/1
  Bus Selector/7 -> Process Noise I=23-6/2  "<XMNSEG>"
  Bus Selector/8 -> Process Noise I=23-7/2  "<XMNSEH>"
  Bus Selector/6 -> Process Noise I=23-5/2  "<XMNSEF>"
  Bus Selector/5 -> Process Noise I=23-4/2  "<XMNSEE>"
  Bus Selector/4 -> Process Noise I=23-3/2  "<XMNSED>"
  Bus Selector/3 -> Process Noise I=23-2/2  "<XMNSEC>"
  Bus Selector/1 -> Process Noise I=23-36/2  "<XMNSEA>"
  XST/1 -> Subsystem/1(XST)
  Subsystem/1(XCMPA) -> Process Noise I=23-36/1
  Subsystem/2(XCMPB) -> Process Noise I=23-1/1
  Subsystem/3(XCMPC) -> Process Noise I=23-2/1
  Subsystem/4(XCMPD) -> Process Noise I=23-3/1
  Subsystem/5("XCMPE ") -> Process Noise I=23-4/1
  Subsystem/6("XCMPF ") -> Process Noise I=23-5/1
  Subsystem/7(XCMPG) -> Process Noise I=23-6/1
  Subsystem/8("XCMPH ") -> Process Noise I=23-7/1
  XMNSE/1 -> Bus Selector/1

== system TEP_Final_NoScript/Subsystem1/Product stream/Composition measurement mol%/Subsystem ==
  XST : Inport
  XMNSE : Inport  Port=2
  Bus Selector : BusSelector  OutputSignals=XMNSEA,XMNSEB,XMNSEC
  Process Noise I=23-1 : mylib/Process Noise I=23-36  SystemSampleTime=-1  VariantActivationTime=update diagram  AllowFlexibleInterface=on  Latency=0  AutoFrameSizeCalculation=off
      settings: SourceProductName=TEP Library
  Process Noise I=23-2 : mylib/Process Noise I=23-36  SystemSampleTime=-1  VariantActivationTime=update diagram  AllowFlexibleInterface=on  Latency=0  AutoFrameSizeCalculation=off
      settings: SourceProductName=TEP Library
  Process Noise I=23-36 : mylib/Process Noise I=23-36  SystemSampleTime=-1  VariantActivationTime=update diagram  AllowFlexibleInterface=on  Latency=0  AutoFrameSizeCalculation=off
      settings: SourceProductName=TEP Library
  Subsystem : Subsystem
  SMEASXA : Outport  VectorParamsAs1DForOutWhenUnconnected=off
  SMEASXB : Outport  Port=2  VectorParamsAs1DForOutWhenUnconnected=off
  SMEASXC : Outport  Port=3  VectorParamsAs1DForOutWhenUnconnected=off
  wires:
  Process Noise I=23-36/1 -> SMEASXA/1
  Process Noise I=23-1/1 -> SMEASXB/1
  Bus Selector/2 -> Process Noise I=23-1/2  "<XMNSEB>"
  Process Noise I=23-2/1 -> SMEASXC/1
  Bus Selector/3 -> Process Noise I=23-2/2  "<XMNSEC>"
  Bus Selector/1 -> Process Noise I=23-36/2  "<XMNSEA>"
  XST/1 -> Subsystem/1(XST)
  Subsystem/1(XCMPA) -> Process Noise I=23-36/1
  Subsystem/2(XCMPB) -> Process Noise I=23-1/1
  Subsystem/3(XCMPC) -> Process Noise I=23-2/1
  XMNSE/1 -> Bus Selector/1

== system TEP_Final_NoScript/Subsystem1/Product stream/Composition measurement mol%/Subsystem1 ==
  XST : Inport
  XMNSE3 : Inport  Port=2
  Bus Selector : BusSelector  OutputSignals=XMNSED,XMNSEE,XMNSEF,XMNSEG,XMNSEH
  Process Noise I=37-{1..4,41} (5 alike) : mylib/Process Noise I=37-41  SystemSampleTime=-1  VariantActivationTime=update diagram  AllowFlexibleInterface=on  Latency=0  AutoFrameSizeCalculation=off
      settings: SourceProductName=TEP Library
  Subsystem : Subsystem
  SMEASXD : Outport  VectorParamsAs1DForOutWhenUnconnected=off
  SMEASXE : Outport  Port=2  VectorParamsAs1DForOutWhenUnconnected=off
  SMEASXF : Outport  Port=3  VectorParamsAs1DForOutWhenUnconnected=off
  SMEASXG : Outport  Port=4  VectorParamsAs1DForOutWhenUnconnected=off
  SMEASXH : Outport  Port=5  VectorParamsAs1DForOutWhenUnconnected=off
  wires:
  Process Noise I=37-41/1 -> SMEASXD/1
  Bus Selector/1 -> Process Noise I=37-41/2  "<XMNSED>"
  Process Noise I=37-1/1 -> SMEASXE/1
  Bus Selector/2 -> Process Noise I=37-1/2  "<XMNSEE>"
  Process Noise I=37-2/1 -> SMEASXF/1
  Bus Selector/3 -> Process Noise I=37-2/2  "<XMNSEF>"
  Process Noise I=37-3/1 -> SMEASXG/1
  Bus Selector/4 -> Process Noise I=37-3/2  "<XMNSEG>"
  Process Noise I=37-4/1 -> SMEASXH/1
  Bus Selector/5 -> Process Noise I=37-4/2  "<XMNSEH>"
  XST/1 -> Subsystem/1(XST)
  Subsystem/1(XCMPD) -> Process Noise I=37-41/1
  Subsystem/2("XCMPE ") -> Process Noise I=37-1/1
  Subsystem/3("XCMPF ") -> Process Noise I=37-2/1
  Subsystem/4(XCMPG) -> Process Noise I=37-3/1
  Subsystem/5("XCMPH ") -> Process Noise I=37-4/1
  XMNSE3/1 -> Bus Selector/1

== system TEP_Final_NoScript/Subsystem1/Product stream/Flow measurement in kg//h/XMWS Molecular weight of Stream lb//lb-mol ==
  XST : Inport
  Product : Product
  Sum of Elements : Sum  Inputs=+
  "XMW(I) Molecular weight of components lb/lb-mol " : Constant  Value=XMW
  XMWS : Outport  VectorParamsAs1DForOutWhenUnconnected=off
  wires:
  Sum of Elements/1 -> XMWS/1
  Product/1 -> Sum of Elements/1
  XST/1 -> Product/1
  "XMW(I) Molecular weight of components lb/lb-mol "/1 -> Product/2

== system TEP_Final_NoScript/Subsystem1/Purge stream/Flow measurement in kg//h/XMWS Molecular weight of Stream lb//lb-mol ==
  XST : Inport
  Product : Product
  Sum of Elements : Sum  Inputs=+
  "XMW(I) Molecular weight of components lb/lb-mol " : Constant  Value=XMW
  XMWS : Outport  VectorParamsAs1DForOutWhenUnconnected=off
  wires:
  Sum of Elements/1 -> XMWS/1
  Product/1 -> Sum of Elements/1
  XST/1 -> Product/1
  "XMW(I) Molecular weight of components lb/lb-mol "/1 -> Product/2

== system TEP_Final_NoScript/Subsystem1/RCin/Subsystem3/Subsystem ==
  T1 : Inport
  T0 : Inport  Port=2
  Product3 : Product
  Subsystem2 : Subsystem
  Universal gas constant J/molK : Constant  Value=8.314
  h-h0 J/mol : Outport
  wires:
  T1/1 -> Subsystem2/1(T1)
  T0/1 -> Subsystem2/2(T0)
  Subsystem2/1(AT) -> Product3/1
  Universal gas constant J/molK/1 -> Product3/2
  Product3/1 -> h-h0 J/mol/1

== system TEP_Final_NoScript/Subsystem1/RCin/Subsystem3/Subsystem1 ==
  T1 : Inport
  T0 : Inport  Port=2
  P1 : Inport  Port=3
  P0 : Inport  Port=4
  " " : Product
  Add : Sum  Inputs=+-
  Display{1..8} (8 alike) : Display
  Divide : Product  Inputs=*/
  Math Function2 : Math  Operator=log  SignedPower=on
  Product3 : Product  Inputs=3
  Product6 : Product
  Subsystem : Subsystem
  Universal gas constant J/molK : Constant  Value=8.314
  T0(s-s0) J/mol : Outport
  wires:
  T1/1 -> Display6/1, Subsystem/1(T1)
  Subsystem/1(AT) -> Display8/1, Product3/1
  Universal gas constant J/molK/1 -> Product6/1, Product3/2
  T0/1 -> " "/1, Display7/1, Product3/3, Subsystem/2(T0)
  Math Function2/1 -> Display5/1, Product6/2
  Product6/1 -> Display4/1, " "/2
  Divide/1 -> Display2/1, Math Function2/1
  P0/1 -> Divide/2
  P1/1 -> Divide/1
  Product3/1 -> Add/1, Display3/1
  Add/1 -> T0(s-s0) J/mol/1
  " "/1 -> Add/2, Display1/1

== system TEP_Final_NoScript/Subsystem1/RCin/Subsystem3/Subsystem2 ==
  TC : Inport
  Temperature in Kelvin K : Sum
  To Convert °C to K : Constant  Value=273.15
  TK : Outport
  wires:
  TC/1 -> Temperature in Kelvin K/1
  Temperature in Kelvin K/1 -> TK/1
  To Convert °C to K/1 -> Temperature in Kelvin K/2

== system TEP_Final_NoScript/Subsystem1/RCout/Subsystem3/Subsystem ==
  T1 : Inport
  T0 : Inport  Port=2
  Product3 : Product
  Subsystem2 : Subsystem
  Universal gas constant J/molK : Constant  Value=8.314
  h-h0 J/mol : Outport
  wires:
  T1/1 -> Subsystem2/1(T1)
  T0/1 -> Subsystem2/2(T0)
  Subsystem2/1(AT) -> Product3/1
  Universal gas constant J/molK/1 -> Product3/2
  Product3/1 -> h-h0 J/mol/1

== system TEP_Final_NoScript/Subsystem1/RCout/Subsystem3/Subsystem1 ==
  T1 : Inport
  T0 : Inport  Port=2
  P1 : Inport  Port=3
  P0 : Inport  Port=4
  " " : Product
  Add : Sum  Inputs=+-
  Display{1..8} (8 alike) : Display
  Divide : Product  Inputs=*/
  Math Function2 : Math  Operator=log  SignedPower=on
  Product3 : Product  Inputs=3
  Product6 : Product
  Subsystem : Subsystem
  Universal gas constant J/molK : Constant  Value=8.314
  T0(s-s0) J/mol : Outport
  wires:
  T1/1 -> Display6/1, Subsystem/1(T1)
  Subsystem/1(AT) -> Display8/1, Product3/1
  Universal gas constant J/molK/1 -> Product6/1, Product3/2
  T0/1 -> " "/1, Display7/1, Product3/3, Subsystem/2(T0)
  Math Function2/1 -> Display5/1, Product6/2
  Product6/1 -> Display4/1, " "/2
  Divide/1 -> Display2/1, Math Function2/1
  P0/1 -> Divide/2
  P1/1 -> Divide/1
  Product3/1 -> Add/1, Display3/1
  Add/1 -> T0(s-s0) J/mol/1
  " "/1 -> Add/2, Display1/1

== system TEP_Final_NoScript/Subsystem1/RCout/Subsystem3/Subsystem2 ==
  TC : Inport
  Temperature in Kelvin K : Sum
  To Convert °C to K : Constant  Value=273.15
  TK : Outport
  wires:
  TC/1 -> Temperature in Kelvin K/1
  Temperature in Kelvin K/1 -> TK/1
  To Convert °C to K/1 -> Temperature in Kelvin K/2

== system TEP_Final_NoScript/Subsystem1/Reactor feed stream/Composition measurement mol%/Subsystem ==
  XST : Inport
  XMNSE : Inport  Port=2
  XMEAS : Inport  Port=3
  Bus Selector : BusSelector  OutputSignals=XMNSEG,XMNSEH
  Bus Selector1 : BusSelector  OutputSignals=XMEAS(23),XMEAS(24),XMEAS(25),XMEAS(26),XMEAS(27),XMEAS(28)
  Process Noise I=23-6 : mylib/Process Noise I=23-36  SystemSampleTime=-1  VariantActivationTime=update diagram  AllowFlexibleInterface=on  Latency=0  AutoFrameSizeCalculation=off
      settings: SourceProductName=TEP Library
  Process Noise I=23-7 : mylib/Process Noise I=23-36  SystemSampleTime=-1  VariantActivationTime=update diagram  AllowFlexibleInterface=on  Latency=0  AutoFrameSizeCalculation=off
      settings: SourceProductName=TEP Library
  Subsystem : Subsystem
  SMEASXA : Outport  VectorParamsAs1DForOutWhenUnconnected=off
  SMEASXB : Outport  Port=2  VectorParamsAs1DForOutWhenUnconnected=off
  SMEASXC : Outport  Port=3  VectorParamsAs1DForOutWhenUnconnected=off
  SMEASXD : Outport  Port=4  VectorParamsAs1DForOutWhenUnconnected=off
  SMEASXE : Outport  Port=5  VectorParamsAs1DForOutWhenUnconnected=off
  SMEASXF : Outport  Port=6  VectorParamsAs1DForOutWhenUnconnected=off
  SMEASXG : Outport  Port=7  VectorParamsAs1DForOutWhenUnconnected=off
  SMEASXH : Outport  Port=8  VectorParamsAs1DForOutWhenUnconnected=off
  wires:
  Bus Selector1/1 -> SMEASXA/1  "<XMEAS(23)>"
  Bus Selector1/2 -> SMEASXB/1  "<XMEAS(24)>"
  Bus Selector1/3 -> SMEASXC/1  "<XMEAS(25)>"
  Bus Selector1/4 -> SMEASXD/1  "<XMEAS(26)>"
  Bus Selector1/5 -> SMEASXE/1  "<XMEAS(27)>"
  Bus Selector1/6 -> SMEASXF/1  "<XMEAS(28)>"
  Process Noise I=23-6/1 -> SMEASXG/1
  Process Noise I=23-7/1 -> SMEASXH/1
  Bus Selector/1 -> Process Noise I=23-6/2  "<XMNSEG>"
  Bus Selector/2 -> Process Noise I=23-7/2  "<XMNSEH>"
  XST/1 -> Subsystem/1(XST)
  Subsystem/1(XCMPG) -> Process Noise I=23-6/1
  Subsystem/2("XCMPH ") -> Process Noise I=23-7/1
  XMNSE/1 -> Bus Selector/1
  XMEAS/1 -> Bus Selector1/1

== system TEP_Final_NoScript/Subsystem1/Reactor feed stream/Flow measurement in kg//h/XMWS Molecular weight of Stream lb//lb-mol ==
  XST : Inport
  Product : Product
  Sum of Elements : Sum  Inputs=+
  "XMW(I) Molecular weight of components lb/lb-mol " : Constant  Value=XMW
  XMWS : Outport  VectorParamsAs1DForOutWhenUnconnected=off
  wires:
  Sum of Elements/1 -> XMWS/1
  Product/1 -> Sum of Elements/1
  XST/1 -> Product/1
  "XMW(I) Molecular weight of components lb/lb-mol "/1 -> Product/2

== system TEP_Final_NoScript/Subsystem1/Reactor product stream/Composition measurement mol%/Subsystem ==
  XST : Inport
  XMNSE : Inport  Port=2
  Bus Selector : BusSelector  OutputSignals=XMNSEA,XMNSEB,XMNSEC,XMNSED,XMNSEE,XMNSEF,XMNSEG,XMNSEH
  Process Noise I=23-{1..7,36} (8 alike) : mylib/Process Noise I=23-36  SystemSampleTime=-1  VariantActivationTime=update diagram  AllowFlexibleInterface=on  Latency=0  AutoFrameSizeCalculation=off
      settings: SourceProductName=TEP Library
  Subsystem : Subsystem
  SMEASXA : Outport  VectorParamsAs1DForOutWhenUnconnected=off
  SMEASXB : Outport  Port=2  VectorParamsAs1DForOutWhenUnconnected=off
  SMEASXC : Outport  Port=3  VectorParamsAs1DForOutWhenUnconnected=off
  SMEASXD : Outport  Port=4  VectorParamsAs1DForOutWhenUnconnected=off
  SMEASXE : Outport  Port=5  VectorParamsAs1DForOutWhenUnconnected=off
  SMEASXF : Outport  Port=6  VectorParamsAs1DForOutWhenUnconnected=off
  SMEASXG : Outport  Port=7  VectorParamsAs1DForOutWhenUnconnected=off
  SMEASXH : Outport  Port=8  VectorParamsAs1DForOutWhenUnconnected=off
  wires:
  Process Noise I=23-36/1 -> SMEASXA/1
  Process Noise I=23-1/1 -> SMEASXB/1
  Bus Selector/2 -> Process Noise I=23-1/2  "<XMNSEB>"
  Process Noise I=23-2/1 -> SMEASXC/1
  Process Noise I=23-3/1 -> SMEASXD/1
  Process Noise I=23-4/1 -> SMEASXE/1
  Process Noise I=23-5/1 -> SMEASXF/1
  Process Noise I=23-6/1 -> SMEASXG/1
  Process Noise I=23-7/1 -> SMEASXH/1
  Bus Selector/7 -> Process Noise I=23-6/2  "<XMNSEG>"
  Bus Selector/8 -> Process Noise I=23-7/2  "<XMNSEH>"
  Bus Selector/6 -> Process Noise I=23-5/2  "<XMNSEF>"
  Bus Selector/5 -> Process Noise I=23-4/2  "<XMNSEE>"
  Bus Selector/4 -> Process Noise I=23-3/2  "<XMNSED>"
  Bus Selector/3 -> Process Noise I=23-2/2  "<XMNSEC>"
  Bus Selector/1 -> Process Noise I=23-36/2  "<XMNSEA>"
  XST/1 -> Subsystem/1(XST)
  Subsystem/1(XCMPA) -> Process Noise I=23-36/1
  Subsystem/2(XCMPB) -> Process Noise I=23-1/1
  Subsystem/3(XCMPC) -> Process Noise I=23-2/1
  Subsystem/4(XCMPD) -> Process Noise I=23-3/1
  Subsystem/5("XCMPE ") -> Process Noise I=23-4/1
  Subsystem/6("XCMPF ") -> Process Noise I=23-5/1
  Subsystem/7(XCMPG) -> Process Noise I=23-6/1
  Subsystem/8("XCMPH ") -> Process Noise I=23-7/1
  XMNSE/1 -> Bus Selector/1

== system TEP_Final_NoScript/Subsystem1/Reactor product stream/Flow measurement in kg//h/XMWS Molecular weight of Stream lb//lb-mol ==
  XST : Inport
  Product : Product
  Sum of Elements : Sum  Inputs=+
  "XMW(I) Molecular weight of components lb/lb-mol " : Constant  Value=XMW
  XMWS : Outport  VectorParamsAs1DForOutWhenUnconnected=off
  wires:
  Sum of Elements/1 -> XMWS/1
  Product/1 -> Sum of Elements/1
  XST/1 -> Product/1
  "XMW(I) Molecular weight of components lb/lb-mol "/1 -> Product/2

== system TEP_Final_NoScript/Subsystem1/Separator recycle stream/Composition measurement mol%/Subsystem ==
  XST : Inport
  XMNSE : Inport  Port=2
  Bus Selector : BusSelector  OutputSignals=XMNSEA,XMNSEB,XMNSEC,XMNSED,XMNSEE,XMNSEF,XMNSEG,XMNSEH
  Process Noise I=23-{1..7,36} (8 alike) : mylib/Process Noise I=23-36  SystemSampleTime=-1  VariantActivationTime=update diagram  AllowFlexibleInterface=on  Latency=0  AutoFrameSizeCalculation=off
      settings: SourceProductName=TEP Library
  Subsystem : Subsystem
  SMEASXA : Outport  VectorParamsAs1DForOutWhenUnconnected=off
  SMEASXB : Outport  Port=2  VectorParamsAs1DForOutWhenUnconnected=off
  SMEASXC : Outport  Port=3  VectorParamsAs1DForOutWhenUnconnected=off
  SMEASXD : Outport  Port=4  VectorParamsAs1DForOutWhenUnconnected=off
  SMEASXE : Outport  Port=5  VectorParamsAs1DForOutWhenUnconnected=off
  SMEASXF : Outport  Port=6  VectorParamsAs1DForOutWhenUnconnected=off
  SMEASXG : Outport  Port=7  VectorParamsAs1DForOutWhenUnconnected=off
  SMEASXH : Outport  Port=8  VectorParamsAs1DForOutWhenUnconnected=off
  wires:
  Process Noise I=23-36/1 -> SMEASXA/1
  Process Noise I=23-1/1 -> SMEASXB/1
  Bus Selector/2 -> Process Noise I=23-1/2  "<XMNSEB>"
  Process Noise I=23-2/1 -> SMEASXC/1
  Process Noise I=23-3/1 -> SMEASXD/1
  Process Noise I=23-4/1 -> SMEASXE/1
  Process Noise I=23-5/1 -> SMEASXF/1
  Process Noise I=23-6/1 -> SMEASXG/1
  Process Noise I=23-7/1 -> SMEASXH/1
  Bus Selector/7 -> Process Noise I=23-6/2  "<XMNSEG>"
  Bus Selector/8 -> Process Noise I=23-7/2  "<XMNSEH>"
  Bus Selector/6 -> Process Noise I=23-5/2  "<XMNSEF>"
  Bus Selector/5 -> Process Noise I=23-4/2  "<XMNSEE>"
  Bus Selector/4 -> Process Noise I=23-3/2  "<XMNSED>"
  Bus Selector/3 -> Process Noise I=23-2/2  "<XMNSEC>"
  Bus Selector/1 -> Process Noise I=23-36/2  "<XMNSEA>"
  XST/1 -> Subsystem/1(XST)
  Subsystem/1(XCMPA) -> Process Noise I=23-36/1
  Subsystem/2(XCMPB) -> Process Noise I=23-1/1
  Subsystem/3(XCMPC) -> Process Noise I=23-2/1
  Subsystem/4(XCMPD) -> Process Noise I=23-3/1
  Subsystem/5("XCMPE ") -> Process Noise I=23-4/1
  Subsystem/6("XCMPF ") -> Process Noise I=23-5/1
  Subsystem/7(XCMPG) -> Process Noise I=23-6/1
  Subsystem/8("XCMPH ") -> Process Noise I=23-7/1
  XMNSE/1 -> Bus Selector/1

== system TEP_Final_NoScript/Subsystem1/Separator recycle stream/Flow measurement in kg//h/XMWS Molecular weight of Stream lb//lb-mol ==
  XST : Inport
  Product : Product
  Sum of Elements : Sum  Inputs=+
  "XMW(I) Molecular weight of components lb/lb-mol " : Constant  Value=XMW
  XMWS : Outport  VectorParamsAs1DForOutWhenUnconnected=off
  wires:
  Sum of Elements/1 -> XMWS/1
  Product/1 -> Sum of Elements/1
  XST/1 -> Product/1
  "XMW(I) Molecular weight of components lb/lb-mol "/1 -> Product/2

== system TEP_Final_NoScript/Subsystem1/Separator underflow stream/Composition measurement mol%/Subsystem ==
  XST : Inport
  XMNSE : Inport  Port=2
  Bus Selector : BusSelector  OutputSignals=XMNSED,XMNSEE,XMNSEF,XMNSEG,XMNSEH
  Constant : Constant  Value=0
  Constant1 : Constant  Value=0
  Constant2 : Constant  Value=0
  Process Noise I=23-{1..7,36} (8 alike) : mylib/Process Noise I=23-36  SystemSampleTime=-1  VariantActivationTime=update diagram  AllowFlexibleInterface=on  Latency=0  AutoFrameSizeCalculation=off
      settings: SourceProductName=TEP Library
  Subsystem : Subsystem
  SMEASXA : Outport  VectorParamsAs1DForOutWhenUnconnected=off
  SMEASXB : Outport  Port=2  VectorParamsAs1DForOutWhenUnconnected=off
  SMEASXC : Outport  Port=3  VectorParamsAs1DForOutWhenUnconnected=off
  SMEASXD : Outport  Port=4  VectorParamsAs1DForOutWhenUnconnected=off
  SMEASXE : Outport  Port=5  VectorParamsAs1DForOutWhenUnconnected=off
  SMEASXF : Outport  Port=6  VectorParamsAs1DForOutWhenUnconnected=off
  SMEASXG : Outport  Port=7  VectorParamsAs1DForOutWhenUnconnected=off
  SMEASXH : Outport  Port=8  VectorParamsAs1DForOutWhenUnconnected=off
  wires:
  Process Noise I=23-36/1 -> SMEASXA/1
  Process Noise I=23-1/1 -> SMEASXB/1
  Process Noise I=23-2/1 -> SMEASXC/1
  Process Noise I=23-3/1 -> SMEASXD/1
  Process Noise I=23-4/1 -> SMEASXE/1
  Process Noise I=23-5/1 -> SMEASXF/1
  Process Noise I=23-6/1 -> SMEASXG/1
  Process Noise I=23-7/1 -> SMEASXH/1
  Bus Selector/4 -> Process Noise I=23-6/2  "<XMNSEG>"
  Bus Selector/5 -> Process Noise I=23-7/2  "<XMNSEH>"
  Bus Selector/3 -> Process Noise I=23-5/2  "<XMNSEF>"
  Bus Selector/2 -> Process Noise I=23-4/2  "<XMNSEE>"
  Bus Selector/1 -> Process Noise I=23-3/2  "<XMNSED>"
  XST/1 -> Subsystem/1(XST)
  Subsystem/1(XCMPA) -> Process Noise I=23-36/1
  Subsystem/2(XCMPB) -> Process Noise I=23-1/1
  Subsystem/3(XCMPC) -> Process Noise I=23-2/1
  Subsystem/4(XCMPD) -> Process Noise I=23-3/1
  Subsystem/5("XCMPE ") -> Process Noise I=23-4/1
  Subsystem/6("XCMPF ") -> Process Noise I=23-5/1
  Subsystem/7(XCMPG) -> Process Noise I=23-6/1
  Subsystem/8("XCMPH ") -> Process Noise I=23-7/1
  XMNSE/1 -> Bus Selector/1
  Constant/1 -> Process Noise I=23-36/2
  Constant1/1 -> Process Noise I=23-1/2
  Constant2/1 -> Process Noise I=23-2/2

== system TEP_Final_NoScript/Subsystem1/Separator underflow stream/Flow measurement in kg//h/XMWS Molecular weight of Stream lb//lb-mol ==
  XST : Inport
  Product : Product
  Sum of Elements : Sum  Inputs=+
  "XMW(I) Molecular weight of components lb/lb-mol " : Constant  Value=XMW
  XMWS : Outport  VectorParamsAs1DForOutWhenUnconnected=off
  wires:
  Sum of Elements/1 -> XMWS/1
  Product/1 -> Sum of Elements/1
  XST/1 -> Product/1
  "XMW(I) Molecular weight of components lb/lb-mol "/1 -> Product/2
